simulink model "CA2_model"  (R2023b)
settings: Solver=VariableStepAuto  StartTime=0.0  StopTime=300  RelTol=1e-3
undefined symbols (not defined in the file): Kc, TI
settings Model: Creator=99551  LastModifiedBy=99551

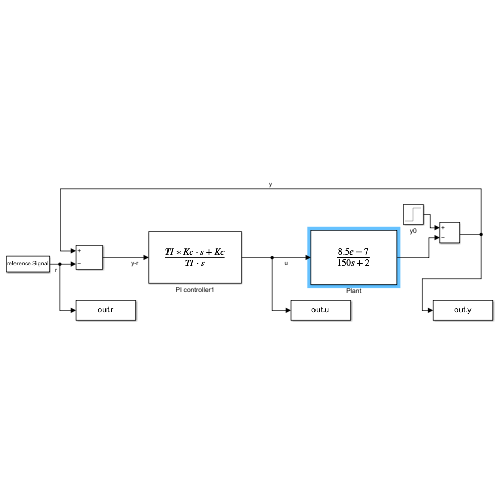
[thumbnail: Simulink's stored preview of the top-level diagram]
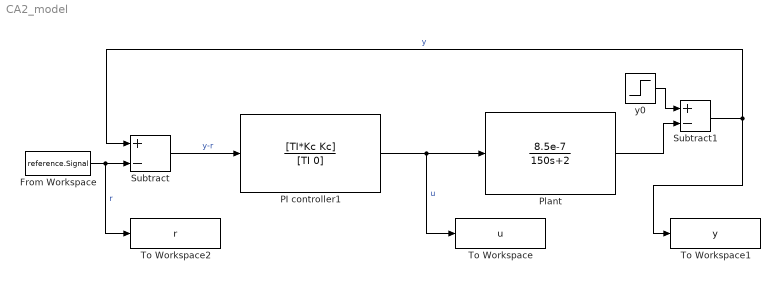
== system CA2_model ==
  From Workspace : FromWorkspace  VariableName=reference.Signal  SampleTime=0.01
  PI controller1 : TransferFcn  Numerator=[TI*Kc Kc]  Denominator=[TI 0]
  Plant : TransferFcn  Numerator=[8.5e-7]  Denominator=[150 2]
  Subtract : Sum  Inputs=+-
  Subtract1 : Sum  Inputs=+-
  To Workspace : ToWorkspace  VariableName=u  SaveFormat=Timeseries  SampleTime=0.01
  To Workspace1 : ToWorkspace  VariableName=y  SaveFormat=Timeseries  SampleTime=0.01
  To Workspace2 : ToWorkspace  VariableName=r  SaveFormat=Timeseries  SampleTime=0.01
  y0 : Step  Time=0  Before=11000  After=11000
  wires:
  PI controller1/1 -> To Workspace/1, Plant/1  "u"
  Subtract/1 -> PI controller1/1  "y-r"
  From Workspace/1 -> To Workspace2/1, Subtract/2  "r"
  Plant/1 -> Subtract1/2
  y0/1 -> Subtract1/1
  Subtract1/1 -> Subtract/1, To Workspace1/1  "y"
